simulink model "VAV02"  (R2018a)
settings: Solver=VariableStepAuto  StartTime=0.0  StopTime=2000  RelTol=1e-3
InitFcn:
  | parameter_und_enverioment
values from neighbouring files (symbols this model uses):
  A = C\A    [parameter_und_enverioment_8_3.m]
  B = C\B    [parameter_und_enverioment_8_3.m]
  Ct = [1,0,0,0,0,0 ... (first row only)    [parameter_und_enverioment_8_3.m]
  U = [Tout;Tsa;Qla;Msa]    [parameter_und_enverioment_8_3.m]
  X = [Tin;0;0;0;0;Min]    [parameter_und_enverioment_8_3.m]
settings Model: Creator=19819  LastModifiedBy=19819
settings DataIOCC: ReturnWorkspaceOutputs=on
settings DebuggingCC: UnconnectedInputMsg=none  UnconnectedOutputMsg=none  UnconnectedLineMsg=none  SFMachineParentedDataDiag=error
settings SFSimCC: SimUseLocalCustomCode=on
settings RTWCC: RTWUseLocalCustomCode=on

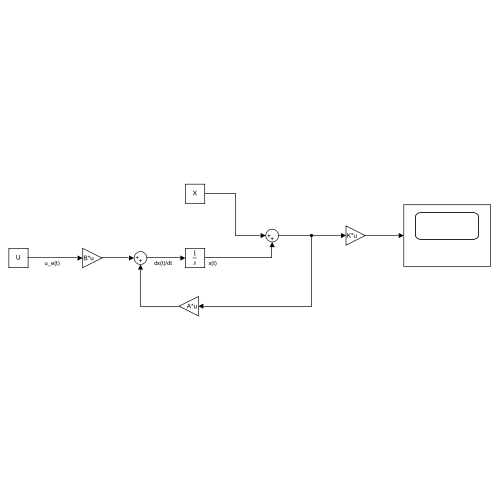
[thumbnail: Simulink's stored preview of the top-level diagram]
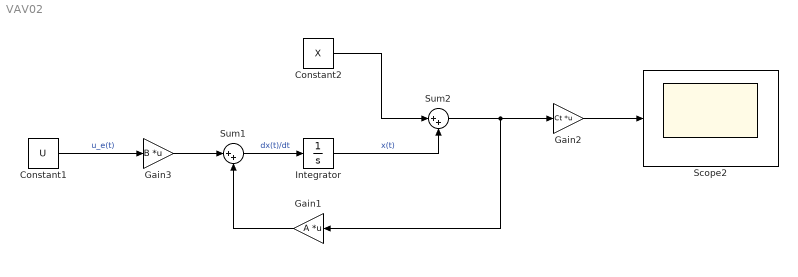
== system VAV02 ==
  Constant1 : Constant  Value=U
  Constant2 : Constant  Value=X
  Gain1 : Gain  Gain=A  Multiplication=Matrix(K*u)
  Gain2 : Gain  Gain=Ct  Multiplication=Matrix(K*u)
  Gain3 : Gain  Gain=B  Multiplication=Matrix(K*u)
  Integrator : Integrator
  Scope2 : Scope
  Sum1 : Sum  Inputs=|++
  Sum2 : Sum  Inputs=|++
  wires:
  Gain1/1 -> Sum1/2
  Sum1/1 -> Integrator/1  "dx(t)/dt"
  Constant1/1 -> Gain3/1  "u_e(t)"
  Gain3/1 -> Sum1/1
  Constant2/1 -> Sum2/1
  Integrator/1 -> Sum2/2  "x(t)"
  Sum2/1 -> Gain2/1, Gain1/1
  Gain2/1 -> Scope2/1
